simulink model "model_v3"  (R2023b)
settings: Solver=VariableStepAuto  StartTime=0.0  StopTime=100  FixedStep=0.001  RelTol=1
settings Model: Creator=ian20030201  LastModifiedBy=ian20030201
settings SolverCC: MaxConsecutiveZCs=1

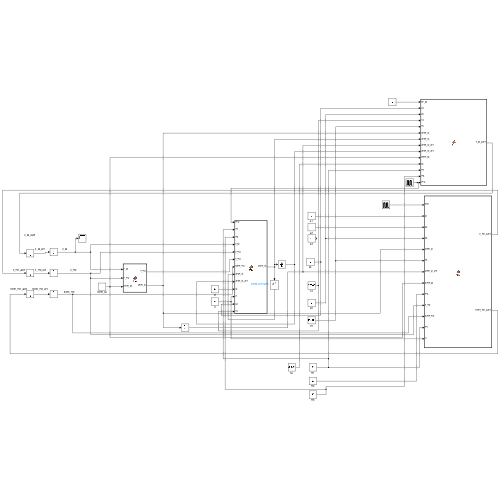
[thumbnail: Simulink's stored preview of the top-level diagram]
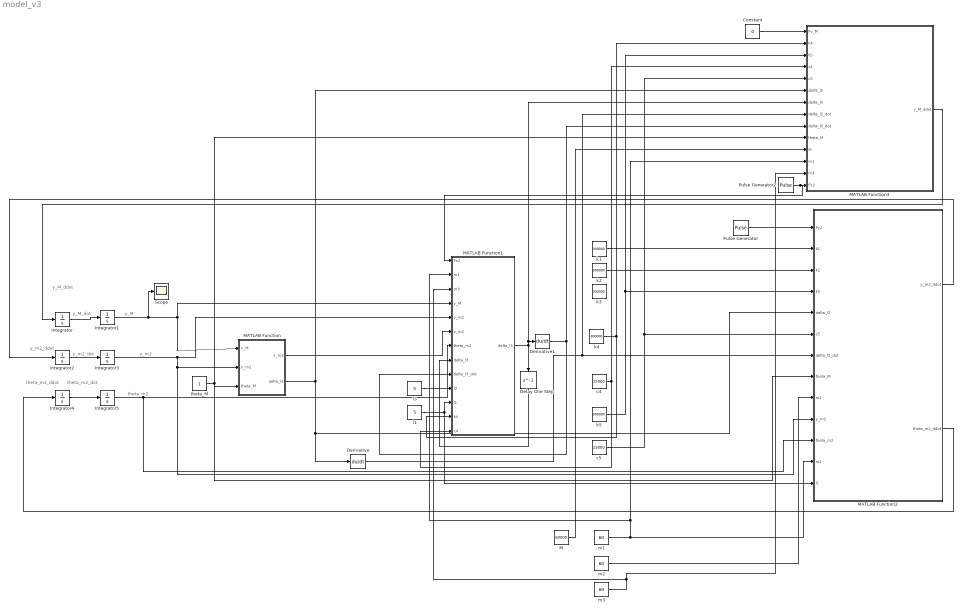
== system model_v3 ==
  note: theta_m2_ddot
  note: y_m2
  note: y_M_ddot
  note: y_M_dot
  note: y_M
  note: y_m2_ddot
  note: y_m2_dot
  note: theta_m2_dot
  note: theta_m2
  Constant : Constant  Value=0
  Delay One Step : Delay  DelayLength=1
  Derivative : Derivative
  Derivative1 : Derivative
  Integrator : Integrator
  Integrator{1..5} (5 alike) : Integrator  InitialCondition=1
  M : Constant  Value=60000
  MATLAB Function : MATLAB Function  TreatAsAtomicUnit=on
  MATLAB Function1 : MATLAB Function  TreatAsAtomicUnit=on
  MATLAB Function2 : MATLAB Function  TreatAsAtomicUnit=on
  MATLAB Function3 : MATLAB Function  TreatAsAtomicUnit=on
  Pulse Generator : DiscretePulseGenerator  PulseType=Time based  Amplitude=200000  Period=100  PulseWidth=5  PhaseDelay=10
  Pulse Generator2 : DiscretePulseGenerator  PulseType=Time based  Amplitude=200000  Period=100  PulseWidth=5  PhaseDelay=10
  Scope : Scope
  c4 : Constant  Value=25000
  c5 : Constant  Value=25000
  k{1..5} (5 alike) : Constant  Value=300000
  l1 : Constant  Value=5
  l3 : Constant  Value=5
  m1 : Constant  Value=60
  m2 : Constant  Value=60
  m3 : Constant  Value=60
  theta_M : Constant
  wires:
  l3/1 -> MATLAB Function1/10(l3)
  l1/1 -> MATLAB Function2/13(l1), MATLAB Function1/11(l1)
  theta_M/1 -> MATLAB Function3/10(theta_M), MATLAB Function2/8(theta_M), MATLAB Function/3(theta_M)
  MATLAB Function3/1(y_M_ddot) -> Integrator/1
  Integrator/1 -> Integrator1/1
  Integrator1/1 -> Scope/1, MATLAB Function1/4(y_M), MATLAB Function/1(y_M)
  MATLAB Function2/1(y_m2_ddot) -> Integrator2/1
  Integrator2/1 -> Integrator3/1
  MATLAB Function2/2(theta_m2_ddot) -> Integrator4/1
  Integrator4/1 -> Integrator5/1
  Integrator3/1 -> MATLAB Function1/5(y_m2), MATLAB Function2/10(y_m2), MATLAB Function/2(y_m2)
  Integrator5/1 -> MATLAB Function2/11(theta_m2), MATLAB Function1/7(theta_m2)
  MATLAB Function/1(x_m2) -> MATLAB Function1/6(x_m2)
  Pulse Generator/1 -> MATLAB Function2/1(Fy2)
  k1/1 -> MATLAB Function2/2(k1)
  k2/1 -> MATLAB Function2/3(k2)
  k5/1 -> MATLAB Function3/3(k5), MATLAB Function2/4(k5)
  c5/1 -> MATLAB Function3/5(c5), MATLAB Function2/6(c5)
  MATLAB Function/2(delta_l2) -> MATLAB Function3/6(delta_l2), Derivative/1, MATLAB Function2/5(delta_l2)
  Derivative/1 -> MATLAB Function3/8(delta_l2_dot), MATLAB Function2/7(delta_l2_dot)
  m1/1 -> MATLAB Function3/12(m1), MATLAB Function1/2(m1), MATLAB Function2/12(m1)
  m2/1 -> MATLAB Function2/9(m2)
  Constant/1 -> MATLAB Function3/1(Fy_M)
  k4/1 -> MATLAB Function3/2(k4), MATLAB Function1/12(k4)
  c4/1 -> MATLAB Function1/13(c4), MATLAB Function3/4(c4)
  Derivative1/1 -> MATLAB Function1/9(delta_l3_dot), MATLAB Function3/9(delta_l3_dot)
  M/1 -> MATLAB Function3/11(M)
  m3/1 -> MATLAB Function1/3(m3), MATLAB Function3/13(m3)
  Pulse Generator2/1 -> MATLAB Function1/1(Fx2), MATLAB Function3/14(Fx2)
  MATLAB Function1/1(delta_l3) -> Delay One Step/1, Derivative1/1, MATLAB Function3/7(delta_l3)
  Delay One Step/1 -> MATLAB Function1/8("delta_l3 ")

== matlab function model_v3/MATLAB Function1 ==
  data: Fx2 input; m1 input; m3 input; y_M input; delta_l3 output; y_m2 input; x_m2 input; theta_m2 input; delta_l3 input; delta_l3_dot input; l3 input; l1 input; k4 input; c4 input
function delta_l3 = fcn(Fx2, m1, m3, y_M, y_m2, x_m2, theta_m2, delta_l3, delta_l3_dot, l3, l1, k4, c4)

%value = (m3*(Fx2/m1)-Fx2)/(k4*delta_l3+c4*delta_l3_dot);
%theta_m3 = asin(max(-1, min(1, value)));
theta_m3 = asin((m3*(Fx2/m1)-Fx2)/(k4*delta_l3+c4*delta_l3_dot));
l3_new = sqrt((l3 * sin(theta_m3) - x_m2)^2 + (l3 * cos(theta_m3) - (y_m2 - l1 * theta_m2) + y_M)^2);
delta_l3 = l3_new - l3;

== matlab function model_v3/MATLAB Function ==
  data: y_M input; x_m2 output; y_m2 input; theta_M input; delta_l2 output
function [x_m2, delta_l2] = fcn(y_M, y_m2, theta_M)

delta_l2 = (y_M - y_m2) / tan(theta_M);
x_m2 = (y_M - y_m2) * tan(theta_M);

== matlab function model_v3/MATLAB Function2 ==
  data: Fy2 input; k1 input; k2 input; y_m2_ddot output; k5 input; theta_m2_ddot output; delta_l2 input; c5 input; delta_l2_dot input; theta_M input; m2 input; y_m2 input; theta_m2 input; m1 input; l1 input
function [y_m2_ddot, theta_m2_ddot] = fcn(Fy2, k1, k2, k5, delta_l2, c5, delta_l2_dot, theta_M, m2, y_m2, theta_m2, m1, l1)

g = 9.81;
y_m2_ddot = Fy2 + (k5 * delta_l2 + c5 * delta_l2_dot) * cos(theta_M) - m2 * g - k2 * y_m2;
theta_m2_ddot = (-k1 * l1 * theta_m2 - k1 * y_m2 - m1 * (g + y_m2_ddot)) / m1;

== matlab function model_v3/MATLAB Function3 ==
  data: Fy_M input; y_M_ddot output; k4 input; k5 input; c4 input; c5 input; delta_l2 input; delta_l3 input; delta_l2_dot input; delta_l3_dot input; theta_M input; M input; m1 input; m3 input; Fx2 input
function y_M_ddot = fcn(Fy_M, k4, k5, c4, c5, delta_l2, delta_l3, delta_l2_dot, delta_l3_dot, theta_M, M, m1, m3, Fx2)

g = 9.81;
%value = (m3*(Fx2/m1)-Fx2)/(k4*delta_l3+c4*delta_l3_dot);
%theta_m3 = asin(max(-1, min(1, value)));
theta_m3 = asin((m3*(Fx2/m1)-Fx2)/(k4*delta_l3+c4*delta_l3_dot));
y_M_ddot = (Fy_M + (k4 * delta_l3 + c4 * delta_l3_dot) * cos(theta_m3) - M * g - (k5 * delta_l2 + c5 * delta_l2_dot) * cos(theta_M)) / M;
